simulink model "sl_drivepoint"  (R2020b)
settings: Solver=ode45  StartTime=0.0  StopTime=15.0  RelTol=1e-3  EnableMultiTasking=on
undefined symbols (not defined in the file or in its folder): xg
libraries: roblocks x1, simulink x1
settings Model: Creator=pic  LastModifiedBy=antonio
settings SolverCC: ZeroCrossAlgorithm=Adaptive
settings DataIOCC: SaveFormat=Array  TimeSaveName=t  OutputSaveName=y
settings OptimizationCC: ExpressionDepthLimit=2147483647  LifeSpan=inf
settings DebuggingCC: UnderspecifiedInitializationDetection=Classic  MergeDetectMultiDrivingBlocksExec=none  IgnoredZcDiagnostic=none  AllowSymbolicDim=off  StateNameClashWarn=warning  SFUnexpectedBacktrackingDiag=warning  SFNoUnconditionalDefaultTransitionDiag=warning  SFExecutionAtInitializationDiag=none  ArithmeticOperatorsInVariantConditions=warning
settings HardwareCC: ProdBitPerPointer=32  ProdBitPerSizeT=32  ProdBitPerPtrDiffT=32  ProdLargestAtomicFloat=None  ProdIntDivRoundTo=Undefined  ProdEndianess=Unspecified  ProdWordSize=32  ProdHWDeviceType=32-bit Generic
settings ModelReferenceCC: PropagateSignalLabelsOutOfModel=off
settings SFSimCC: SimUseLocalCustomCode=off  CustomCodeUndefinedFunction=UseInterfaceOnly
settings RTWCC: RTWUseLocalCustomCode=off
settings CodeAppCC: StateflowObjectComments=on
settings GRTTargetCC: TargetLangStandard=C89/C90 (ANSI)  CombineOutputUpdateFcns=off  GRTInterface=on
settings ConfigComp: CovMetricSettings=dw  CovSaveCumulativeToWorkspaceVar=on  CovSaveSingleToWorkspaceVar=on  CovExternalEMLEnable=off

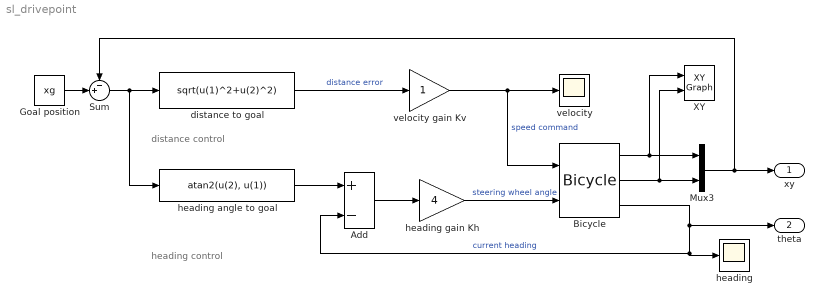
== system sl_drivepoint ==
  note: distance control
  note: heading control
  Add : Sum  Inputs=+-
  Bicycle : roblocks/Vehicles/Bicycle  vlim=1  accel=1  alim=1  steer_rate=Inf  L=1  x0=x0
  Goal position : Constant  Value=xg
  Mux3 : Mux  Inputs=2
  Sum : Sum  Inputs=-+|
  XY : simulink/Sinks/XY Graph  xmin=0  xmax=10  ymin=0  ymax=10  st=-1
  distance to goal : Fcn  Expr=sqrt(u(1)^2+u(2)^2)
  heading : Scope
  heading angle to goal : Fcn  Expr=atan2(u(2), u(1))
  heading gain Kh : Gain  Gain=4
  velocity : Scope
  velocity gain Kv : Gain
  xy : Outport
  "theta " : Outport  Port=2
  wires:
  Bicycle/1 -> Mux3/1, XY/1
  Bicycle/2 -> Mux3/2, XY/2
  Mux3/1 -> Sum/1, xy/1
  Sum/1 -> distance to goal/1, heading angle to goal/1
  distance to goal/1 -> velocity gain Kv/1  "distance error"
  Bicycle/3 -> Add/2, heading/1, "theta "/1  "current heading"
  velocity gain Kv/1 -> Bicycle/1, velocity/1  "speed command"
  Goal position/1 -> Sum/2
  heading gain Kh/1 -> Bicycle/2  "steering wheel angle"
  heading angle to goal/1 -> Add/1
  Add/1 -> heading gain Kh/1
